simulink model "SimplifiedSensorRead"  (R2023a)
settings: Solver=VariableStepAuto  StartTime=0.0  StopTime=inf  RelTol=1e-3
undefined symbols (not defined in the file): LF
libraries: instrumentseriallib x2
settings Model: Creator=karim  LastModifiedBy=karim

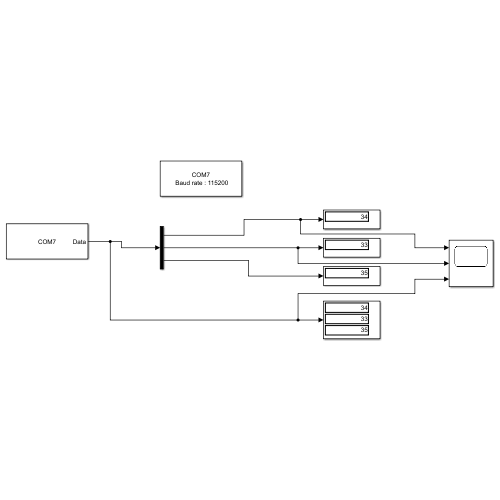
[thumbnail: Simulink's stored preview of the top-level diagram]
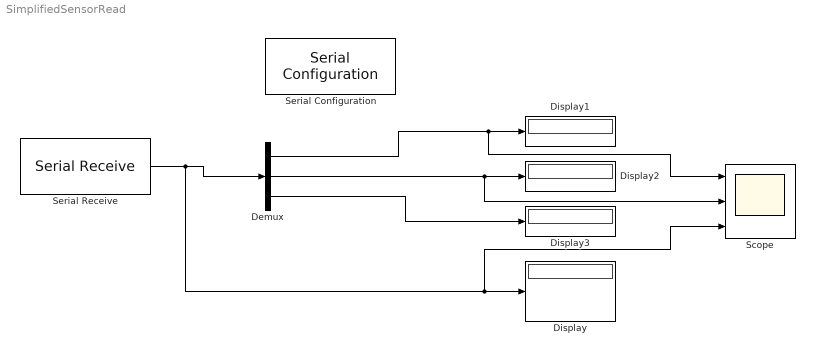
== system SimplifiedSensorRead ==
  Demux : Demux  Outputs=3
  Display{,1..3} (4 alike) : Display
      Display settings: Decimation=3
  Scope : Scope  NumInputPorts=3
  Serial Configuration : instrumentseriallib/Serial Configuration  Priority=-200000  PortSel=COM7  Port=COM7  ComPort=COM7  BaudRate=115200  DataBits=8  Parity=none  StopBits=1  ByteOrder=little-endian  FlowControl=none  Timeout=10  SimulateUsing=Interpreted execution  BlockInModel=on  aMode=1
  Serial Receive : instrumentseriallib/Serial Receive  Priority=1  PortSel=COM7  Port=COM7  ComPort=COM7  DataType=single  SaveDataType=uint8  ToggleHeader=on  Header=[65]  ToggleTerminator=on  Terminator=LF ('\n')  CustomTerminator=[]  InputFormat=Column major  ToggleDataSize=on  DataSize=[1 3]  EnableBlockingMode=on  ActionDataUnavailable=Output last received value  ActionWhenDataUnavailable=Output last received value  CustomValue=0  SampleTime=0.05  SimulateUsing=Interpreted execution  BlockInModel=on  aMode=1
  wires:
  Demux/1 -> Scope/1, Display1/1
  Demux/2 -> Scope/2, Display2/1
  Serial Receive/1 -> Scope/3, Display/1, Demux/1
  Demux/3 -> Display3/1
